simulink model "hr_io_feedback_linearization"  (R2024b)
settings: Solver=ode23s  StartTime=0.0  StopTime=T  RelTol=1e-3
values from neighbouring files (symbols this model uses):
  a = 1    [bifurcation_diagram.m]    (also in equilibria.m; flow.m; flow_analysis.m; linear_analysis.m)
  b = 3    [bifurcation_diagram.m]    (also in equilibria.m; flow.m; flow_analysis.m; linear_analysis.m = linspace(0, 10, 100))
  c = 1    [bifurcation_diagram.m]    (also in equilibria.m; flow.m; flow_analysis.m; linear_analysis.m)
  d = 5    [bifurcation_diagram.m]    (also in equilibria.m; flow.m; flow_analysis.m; linear_analysis.m)
  d_filter = 100    [params.m]
  I = linspace(1.2, 3.5, 1000)    [bifurcation_diagram.m]    (also in equilibria.m = 1.309; flow.m = 1.3059; linear_analysis.m = 2; params.m = 1.28)
  Kd_fbl = 0    [params.m]
  Ki_fbl = 0    [params.m]
  Kp_fbl = 2.5    [params.m]
  r = 0.003    [bifurcation_diagram.m]    (also in equilibria.m; flow.m; flow_analysis.m; linear_analysis.m = 0.001)
  regulation = 0    [params.m]    (also in plot_sim_reg.m = 1; plot_sim_reg_disturbance.m = 1; plot_sim_reg_uncertainties.m = 1; plot_sim_track.m)
  s = 4    [bifurcation_diagram.m]    (also in equilibria.m; flow.m; flow_analysis.m; linear_analysis.m)
  uncertainty = 0    [params.m]    (also in plot_sim_reg.m; plot_sim_reg_disturbance.m; plot_sim_reg_uncertainties.m = 1; plot_sim_track.m)
  x_0 = [0.1; 0.1; 0.1]    [bifurcation_diagram.m]    (also in flow.m = x_0_generic; params.m; plot_sim_track.m = hr_equilibria(a,b,c,d,s,x_r,I); plot_sim_track_disturbance.m = hr_equilibria(a,b,c,d,s,x_r,I))
  x_eq = current_eq(1, j)    [linear_analysis.m]    (also in params.m = eq(1,1); plot_sim_track.m = eq(1,1); plot_sim_track_disturbance.m = eq(1,1); plot_sim_track_uncertainties.m = eq(1,1))
  x_r = -8/5    (= -1.6)    [bifurcation_diagram.m]    (also in equilibria.m; flow.m; flow_analysis.m; linear_analysis.m)
libraries: slpidlib x1
settings Model: Creator=vincip  LastModifiedBy=vincip
settings HardwareCC: ProdBitPerLong=64  ProdHWDeviceType=Intel->x86-64 (Linux 64)

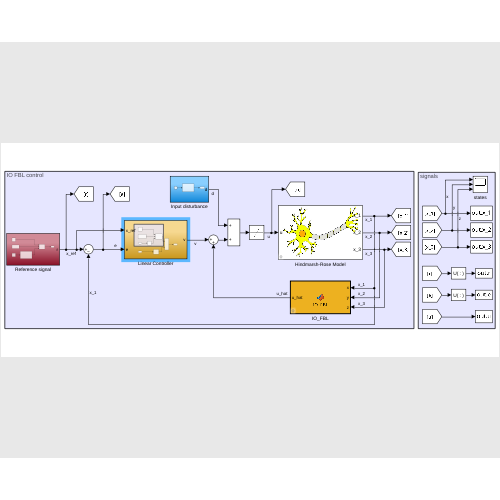
[thumbnail: Simulink's stored preview of the top-level diagram]
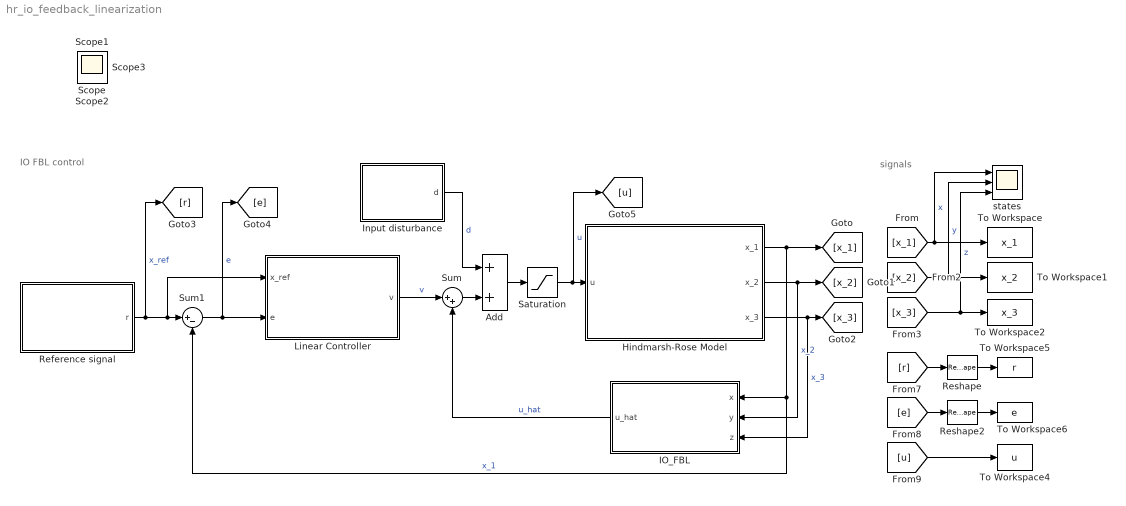
== system hr_io_feedback_linearization ==
  note: signals
  note: IO FBL control
  Add : Sum
  Hindmarsh-Rose Model : Subsystem  mask{a=a, b=b, c=c, d=d, r=r, s=s, x_r=x_r, I=I, x_0=x_0, uncertainty=uncertainty}
      mask DialogControl DescTextVar Prompt: Hindmarsh-Rose Neuronal Model with an external input u
      mask Display:
      | image('figures/neuron.jpg');
      | port_label('input', 1, 'u');
      | port_label('output', 1, 'x_1');
      | port_label('output', 2, 'x_2');
      | port_label('output', 3, 'x_3');
  IO_FBL : MATLAB Function  TreatAsAtomicUnit=on  mask{a=a, b=b, I=I}
  Input disturbance : Subsystem
  Linear Controller : Subsystem
  Reference signal : Subsystem
  Reshape : Reshape
  Reshape2 : Reshape
  Saturation : Saturate  UpperLimit=10  LowerLimit=-10
  Sum : Sum  Inputs=|++
  Sum1 : Sum  Inputs=|+-
  To Workspace : ToWorkspace  VariableName=x_1  SaveFormat=Timeseries  SampleTime=-1
  To Workspace1 : ToWorkspace  VariableName=x_2  SaveFormat=Timeseries  SampleTime=-1
  To Workspace2 : ToWorkspace  VariableName=x_3  SaveFormat=Timeseries  SampleTime=-1
  To Workspace4 : ToWorkspace  VariableName=u  SaveFormat=Timeseries  SampleTime=-1
  To Workspace5 : ToWorkspace  VariableName=r  SaveFormat=Timeseries  SampleTime=-1
  To Workspace6 : ToWorkspace  VariableName=e  SaveFormat=Timeseries  SampleTime=-1
  states : Scope  NumInputPorts=3
  Scope{,1..3} (4 alike) : Scope
  wires:
  Sum1/1 -> Linear Controller/2(e), [e]  "e"
  IO_FBL/1(u_hat) -> Sum/2  "u_hat"
  Sum/1 -> Add/2
  Reshape/1 -> To Workspace5/1
  Reference signal/1(r) -> [r], Linear Controller/1(x_ref), Sum1/1  "x_ref"
  [x_1] -> states/1, To Workspace/1  "x"
  Hindmarsh-Rose Model/2(x_2) -> [x_2], IO_FBL/2(y)  "x_2"
  Hindmarsh-Rose Model/3(x_3) -> IO_FBL/3(z), [x_3]  "x_3"
  [x_2] -> states/2, To Workspace1/1  "y"
  [x_3] -> states/3, To Workspace2/1  "z"
  Hindmarsh-Rose Model/1(x_1) -> [x_1], Sum1/2, IO_FBL/1(x)  "x_1"
  [r] -> Reshape/1
  Reshape2/1 -> To Workspace6/1
  [e] -> Reshape2/1
  [u] -> To Workspace4/1
  Saturation/1 -> [u], Hindmarsh-Rose Model/1(u)  "u"
  Add/1 -> Saturation/1
  Linear Controller/1(v) -> Sum/1  "v"
  Input disturbance/1(d) -> Add/1  "d"

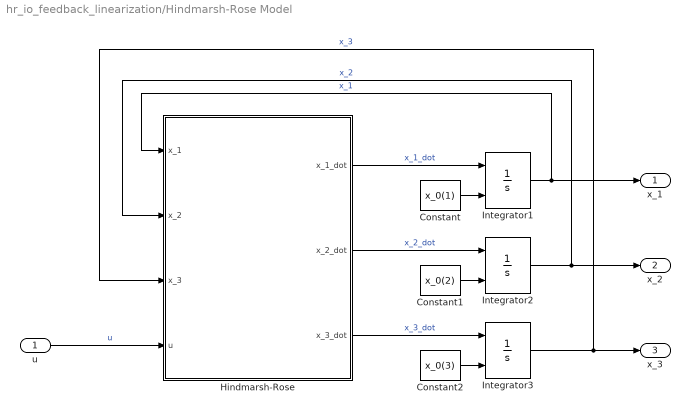
== system hr_io_feedback_linearization/Hindmarsh-Rose Model ==
  u : Inport
  Constant : Constant  Value=x_0(1)
  Constant1 : Constant  Value=x_0(2)
  Constant2 : Constant  Value=x_0(3)
  Hindmarsh-Rose : MATLAB Function  TreatAsAtomicUnit=on
  Integrator1 : Integrator  InitialConditionSource=external  InitialCondition=x_0
  Integrator2 : Integrator  InitialConditionSource=external  InitialCondition=x_0
  Integrator3 : Integrator  InitialConditionSource=external  InitialCondition=x_0
  x_1 : Outport
  x_2 : Outport  Port=2
  x_3 : Outport  Port=3
  wires:
  Hindmarsh-Rose/2(x_2_dot) -> Integrator2/1  "x_2_dot"
  Integrator1/1 -> Hindmarsh-Rose/1(x_1), x_1/1  "x_1"
  Hindmarsh-Rose/3(x_3_dot) -> Integrator3/1  "x_3_dot"
  Integrator3/1 -> x_3/1, Hindmarsh-Rose/3(x_3)  "x_3"
  u/1 -> Hindmarsh-Rose/4(u)  "u"
  Hindmarsh-Rose/1(x_1_dot) -> Integrator1/1  "x_1_dot"
  Integrator2/1 -> Hindmarsh-Rose/2(x_2), x_2/1  "x_2"
  Constant/1 -> Integrator1/2
  Constant1/1 -> Integrator2/2
  Constant2/1 -> Integrator3/2

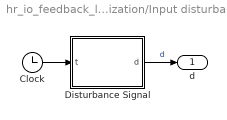
== system hr_io_feedback_linearization/Input disturbance ==
  Clock : Clock
  Disturbance Signal : MATLAB Function  TreatAsAtomicUnit=on
  d : Outport
  wires:
  Clock/1 -> Disturbance Signal/1(t)
  Disturbance Signal/1(d) -> d/1  "d"

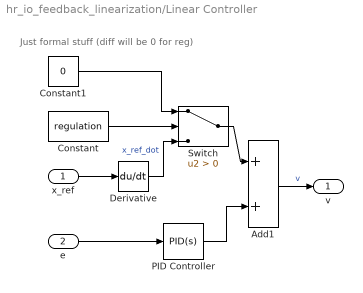
== system hr_io_feedback_linearization/Linear Controller ==
  note: Just formal stuff (diff will be 0 for reg)
  x_ref : Inport
  e : Inport  Port=2
  Add1 : Sum
  Constant : Constant  Value=regulation
  Constant1 : Constant  Value=0
  Derivative : Derivative
  PID Controller : slpidlib/PID Controller  Controller=PID  Form=Parallel  TimeDomain=Continuous-time  UseExternalTs=off  SampleTime=-1  IntegratorMethod=Forward Euler  FilterMethod=Forward Euler  ControllerParametersSource=internal  P=Kp_fbl  I=Ki_fbl  UseKiTs=off  D=Kd_fbl  UseExternalDerivativeSource=off  N=d_filter  UseFilter=on  TunerSelectOption=Transfer Function Based (PID Tuner App)  InitialConditionSource=internal  InitialConditionForIntegrator=0  InitialConditionForFilter=0  DifferentiatorICPrevScaledInput=0  ExternalReset=none  TrackingMode=off  Kt=1  LimitOutput=off  SatLimitsSource=internal  UpperSaturationLimit=inf  LowerSaturationLimit=-inf  LinearizeAsGain=on  AntiWindupMode=none  Kb=1  LimitIntegrator=off  UpperIntegratorSaturationLimit=inf  LowerIntegratorSaturationLimit=-inf  POutMin=[]  POutMax=[]  IOutMin=[]  IOutMax=[]  DOutMin=[]  DOutMax=[]  NOutMin=[]  NOutMax=[]  SumOutMin=[]  SumOutMax=[]  SaturationOutMin=[]  SaturationOutMax=[]  PParamMin=[]  PParamMax=[]  IParamMin=[]  IParamMax=[]  DParamMin=[]  DParamMax=[]  NParamMin=[]  NParamMax=[]  KbParamMin=[]  KbParamMax=[]  KtParamMin=[]  KtParamMax=[]  KbOutMin=[]  KbOutMax=[]  KtOutMin=[]  KtOutMax=[]  IntegratorOutMin=[]  IntegratorOutMax=[]  FilterOutMin=[]  FilterOutMax=[]  SumI1OutMin=[]  SumI1OutMax=[]  SumI2OutMin=[]  SumI2OutMax=[]  SumI3OutMin=[]  SumI3OutMax=[]  SumI4OutMin=[]  SumI4OutMax=[]  SumDOutMin=[]  SumDOutMax=[]  DifferentiatorOutMin=[]  DifferentiatorOutMax=[]  FilterDiffOutCoefMin=[]  FilterDiffOutCoefMax=[]  ReciprocalOutMin=[]  ReciprocalOutMax=[]  SumDenOutMin=[]  SumDenOutMax=[]  SumNumOutMin=[]  SumNumOutMax=[]  DivideOutMin=[]  DivideOutMax=[]  UdiffTsProdOutMin=[]  UdiffTsProdOutMax=[]  NTsProdOutMin=[]  NTsProdOutMax=[]  UintegralTsProdOutMin=[]  UintegralTsProdOutMax=[]  UngainTsProdOutMin=[]  UngainTsProdOutMax=[]  ClampingZeroOutDataTypeStr=Inherit: Inherit via back propagation  ClampingZeroOutMin=[]  ClampingZeroOutMax=[]  FilterDenConstantOutDataTypeStr=Inherit: Inherit via back propagation  FilterDenConstantOutMin=[]  FilterDenConstantOutMax=[]  PCopyOutDataTypeStr=Inherit: Inherit via back propagation  PCopyOutMin=[]  PCopyOutMax=[]  NCopyOutDataTypeStr=Inherit: Inherit via back propagation  NCopyOutMin=[]  NCopyOutMax=[]  IntegratorContinuousStateAttributes=''  IntegratorStateMustResolveToSignalObject=off  IntegratorRTWStateStorageClass=Auto  FilterContinuousStateAttributes=''  FilterStateMustResolveToSignalObject=off  FilterRTWStateStorageClass=Auto  ParallelPVariant=InternalParameters  IdealPVariant=Disabled  IVariant=InternalParameters  DVariant=InternalParameters  IntegratorVariant=Continuous  SatVariant=Disabled  AWVariant=Passthrough  PCopyVariant=Disabled  TRVariant=Disabled  FdbkBlocksVariant=Forward  IdealPFdbkVariant=Disabled  SatFdbkVariant=Disabled  DerivativeFilterVariant=ContFilter  NVariant=InternalParameters  NCopyVariant=Disabled  FilterICVariant=InternalICsFilter  IntegratorICVariant=InternalICs  ExternalResetVariant=Disabled  TRSumVariant=Passthrough  SumFdbkVariant=Disabled  SumVariant=Sum_PID  TsampFilterVariant=InternalTs  TsampNgainVariant=Passthrough  TsampIntegralVariant=Disabled_SignalSpec  ExternalSaturationOutDataTypeStr=Inherit: Same as second input  DerivativeSourceVariant=ErrorSignal  PreIntVariant=InternalPreInt
  Switch : Switch  Criteria=u2 > Threshold  SaturateOnIntegerOverflow=off  InputSameDT=off
  v : Outport
  wires:
  Constant/1 -> Switch/2
  PID Controller/1 -> Add1/2
  Derivative/1 -> Switch/3  "x_ref_dot"
  e/1 -> PID Controller/1
  x_ref/1 -> Derivative/1
  Constant1/1 -> Switch/1
  Switch/1 -> Add1/1
  Add1/1 -> v/1  "v"

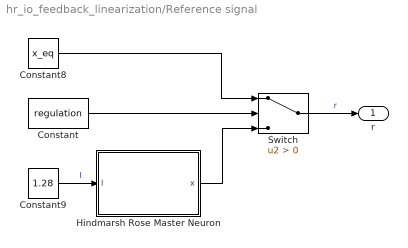
== system hr_io_feedback_linearization/Reference signal ==
  Constant : Constant  Value=regulation
  Constant8 : Constant  Value=x_eq
  Constant9 : Constant  Value=1.28
  Hindmarsh Rose Master Neuron : Subsystem  mask{a=a, b=b, c=c, d=d, r=r, s=s, x_r=x_r, x_0=x_0}
      mask DialogControl DescTextVar Prompt: Hindmarsh-Rose Master neuronal model
      mask Display:
      | disp('Hindmarsh-Rose\nMaster Neuron');
      | port_label('output', 1, 'x');
      | port_label('input', 1, 'I');
  Switch : Switch  Criteria=u2 > Threshold  SaturateOnIntegerOverflow=off  InputSameDT=off
  r : Outport
  wires:
  Hindmarsh Rose Master Neuron/1(x) -> Switch/3
  Constant9/1 -> Hindmarsh Rose Master Neuron/1(I)  "I"
  Constant/1 -> Switch/2
  Constant8/1 -> Switch/1
  Switch/1 -> r/1  "r"

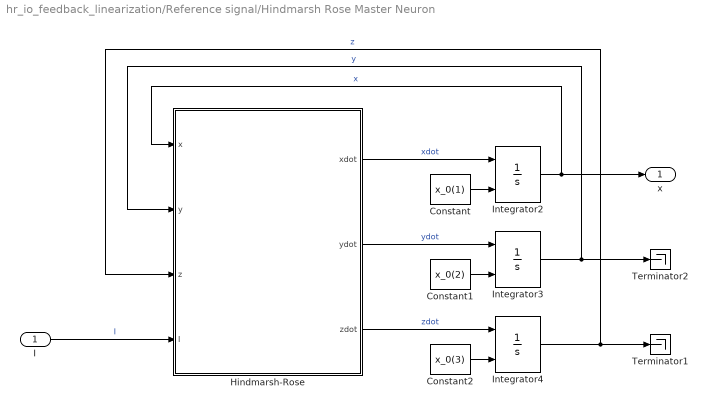
== system hr_io_feedback_linearization/Reference signal/Hindmarsh Rose Master Neuron ==
  I : Inport
  Constant : Constant  Value=x_0(1)
  Constant1 : Constant  Value=x_0(2)
  Constant2 : Constant  Value=x_0(3)
  Hindmarsh-Rose : MATLAB Function  TreatAsAtomicUnit=on
  Integrator2 : Integrator  InitialConditionSource=external  InitialCondition=x_0
  Integrator3 : Integrator  InitialConditionSource=external  InitialCondition=x_0
  Integrator4 : Integrator  InitialConditionSource=external  InitialCondition=x_0
  Terminator1 : Terminator
  Terminator2 : Terminator
  x : Outport
  wires:
  Constant1/1 -> Integrator3/2
  Constant/1 -> Integrator2/2
  Hindmarsh-Rose/2(ydot) -> Integrator3/1  "ydot"
  Constant2/1 -> Integrator4/2
  Integrator4/1 -> Hindmarsh-Rose/3(z), Terminator1/1  "z"
  Integrator2/1 -> Hindmarsh-Rose/1(x), x/1  "x"
  Hindmarsh-Rose/3(zdot) -> Integrator4/1  "zdot"
  Integrator3/1 -> Hindmarsh-Rose/2(y), Terminator2/1  "y"
  I/1 -> Hindmarsh-Rose/4(I)  "I"
  Hindmarsh-Rose/1(xdot) -> Integrator2/1  "xdot"

== matlab function hr_io_feedback_linearization/IO_FBL ==
  data: x input; y input; z input; u_hat output; a parameter; b parameter; I parameter
function u_hat = IO_FBL(x, y, z, a, b, I)
    % u = 1/L_g(h) (v - L_f(h))
    % u_hat = - L_f(h)/L_g(h)
    u_hat = - y + a*x^3 - b*x^2 + z - I;

== matlab function hr_io_feedback_linearization/Input disturbance/Disturbance Signal ==
  data: d output; t input; choice parameter
function d = disturbance(t, choice)
% Select input disturbance based on the choice parameter
ampl = 0.5;
w = 2*pi * 0.2;
if choice == 1
    d = ampl * sin(w * t);
elseif choice == 2
    if t >= 1.0
        d = 1.0;
    else 
        d = 0.0;
    end
else
    d = 0;
end

== matlab function hr_io_feedback_linearization/Hindmarsh-Rose Model/Hindmarsh-Rose ==
  data: x_1 input; x_2 input; x_3 input; u input; x_1_dot output; x_2_dot output; x_3_dot output; a parameter; b parameter; c parameter; d parameter; s parameter; r parameter; x_r parameter; I parameter; uncertainty parameter
function [x_1_dot, x_2_dot, x_3_dot]  = hrindmarsh_rose_model(x_1, x_2, x_3, ...
    u, a, b, c, d, s, r, x_r, I, uncertainty)
    % potential uncertainty
    delta = 0.1;
    if uncertainty == 1
        a_real = a*(1 + delta);
        b_real = b*(1 + delta);
        c_real = c*(1 + delta);
        d_real = d*(1 + delta);
    else
        a_real = a;
        b_real = b;
        c_real = c;
        d_real = d;
    end
    % Neuronal model - Hindmarsh Rose
    x_1_dot = x_2 - a_real*x_1^3 + b_real*x_1^2 - x_3 + I + u;
    x_2_dot = c_real - d_real*x_1^2 - x_2;
    x_3_dot = r*(s*(x_1 - x_r) - x_3);

== matlab function hr_io_feedback_linearization/Reference signal/Hindmarsh Rose Master Neuron/Hindmarsh-Rose ==
  data: x input; y input; z input; xdot output; ydot output; zdot output; a parameter; b parameter; c parameter; d parameter; s parameter; r parameter; x_r parameter; I input
function [xdot, ydot, zdot]  = hrindmarsh_rose_model(x, y, z, a, b, c, d, s, r, x_r, I)
    % Neuronal model - Hindmarsh Rose
    xdot = y - a*x^3 + b*x^2 - z + I;
    ydot = c - d*x^2 - y;
    zdot = r*(s*(x - x_r) - z);
